simulink model "smart_watering_system"  (R2026a)
settings: Solver=FixedStepAuto  EnableMultiTasking=on
libraries: simulink x1, raspberrypiCommlib x1
settings Model: ExtModeTrigDuration=2  Creator=aradskn  LastModifiedBy=manoj
settings SolverCC: PositivePriorityOrder=on
settings OptimizationCC: MaxStackSize=200000
settings HardwareCC: ProdLargestAtomicInteger=Long  ProdLargestAtomicFloat=Double  ProdHWDeviceType=ARM Compatible->ARM Cortex-A (32-bit)
settings RTWCC: SystemTargetFile=ert.tlc  HardwareBoard=Raspberry Pi  TLCOptions="-aInlineSetEventsForThisBaseRateFcn=TLC_FALSE -aSuppressMultiTaskScheduler=TLC_FALSE  -aRateBasedStepFcn=0"  Toolchain=GNU GCC RPIUtils  BuildConfiguration=Faster Runs  Description=Embedded Coder
settings ERTTargetCC: ExtModeTransport=2.0  DynamicArrayContainerType=coder::array  SupportVariableSizeSignals=on

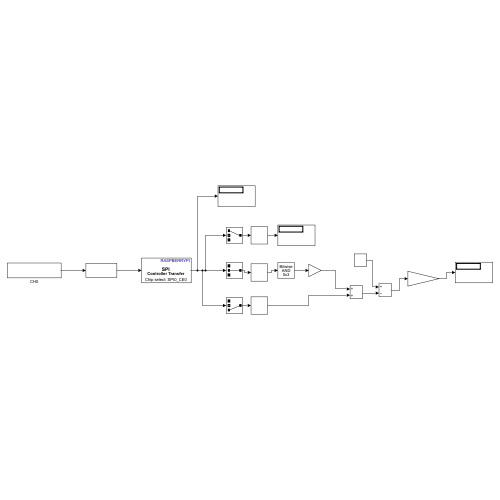
[thumbnail: Simulink's stored preview of the top-level diagram]
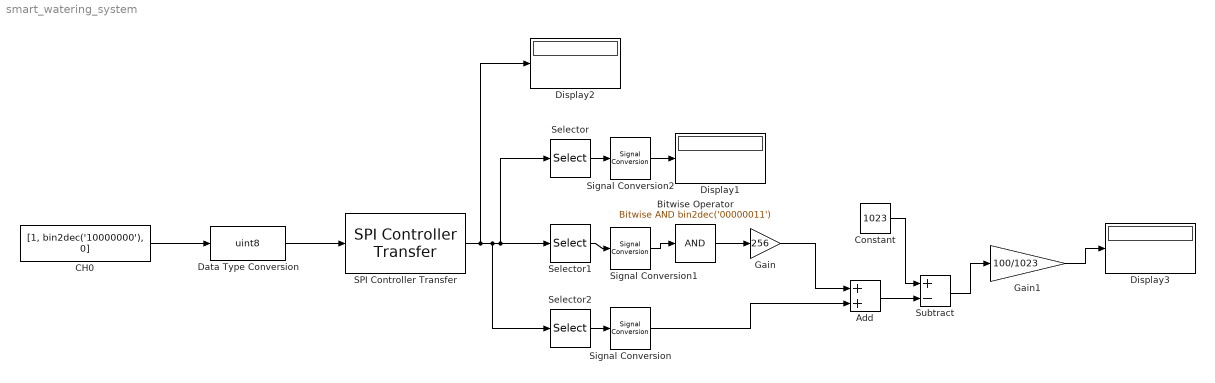
== system smart_watering_system ==
  Add : Sum
  Bitwise Operator : simulink/Logic and Bit Operations/Bitwise Operator  logicop=AND  UseBitMask=on  BitMask=bin2dec('00000011')  BitMaskRealWorld=Stored Integer
  CH0 : Constant  Value=[1, bin2dec('10000000'), 0]
  Constant : Constant  Value=1023
  Data Type Conversion : DataTypeConversion  OutDataTypeStr=uint8  SaturateOnIntegerOverflow=off  RndMeth=Floor
  Display1 : Display
      settings: Format=hex (Stored Integer)
  Display2 : Display
  Display3 : Display
  Gain : Gain  Gain=256
  Gain1 : Gain  Gain=100/1023
  SPI Controller Transfer : raspberrypiCommlib/SPI Controller Transfer  BoardProperty=Pi 4 Model B  SSPin=SPI0_CE0  SPIModule=uint32(0)  Mode=Master  BusSpeed=1000000  Pin=uint32(0)  FirstBitToTransfer=Most significant bit (MSB)  ClockMode=0  BlockFunction=Transfer  RegisterAddress=0  OutputDataType=int8  OutputDataLength=1
  Selector : Selector  InputPortWidth=3  IndexOptions=Index vector (dialog)  Indices=1  OutputSizes=1
  Selector1 : Selector  InputPortWidth=3  IndexOptions=Index vector (dialog)  Indices=2  OutputSizes=1
  Selector2 : Selector  InputPortWidth=3  IndexOptions=Index vector (dialog)  Indices=3  OutputSizes=1
  Signal Conversion : SignalConversion  OverrideOpt=off
  Signal Conversion1 : SignalConversion  OverrideOpt=off
  Signal Conversion2 : SignalConversion  OverrideOpt=off
  Subtract : Sum  Inputs=+-
  wires:
  Selector2/1 -> Signal Conversion/1
  CH0/1 -> Data Type Conversion/1
  Data Type Conversion/1 -> SPI Controller Transfer/1
  Signal Conversion2/1 -> Display1/1
  Selector1/1 -> Signal Conversion1/1
  SPI Controller Transfer/1 -> Display2/1, Selector2/1, Selector/1, Selector1/1
  Selector/1 -> Signal Conversion2/1
  Signal Conversion1/1 -> Bitwise Operator/1
  Bitwise Operator/1 -> Gain/1
  Gain/1 -> Add/1
  Signal Conversion/1 -> Add/2
  Add/1 -> Subtract/2
  Constant/1 -> Subtract/1
  Subtract/1 -> Gain1/1
  Gain1/1 -> Display3/1
